simulink model "Reporting_assignment2"  (R2023b)
settings: Solver=VariableStepAuto  StartTime=0.0  StopTime=2.5  RelTol=1e-3
undefined symbols (not defined in the file): Bm, c1, delta, E, eta, Izzg1, J, Ke, Kp, Kt, La, m1, N, r1, Ra, Td, Ti
settings Model: SimulationMode=accelerator  Creator=Naoki  LastModifiedBy=Naoki

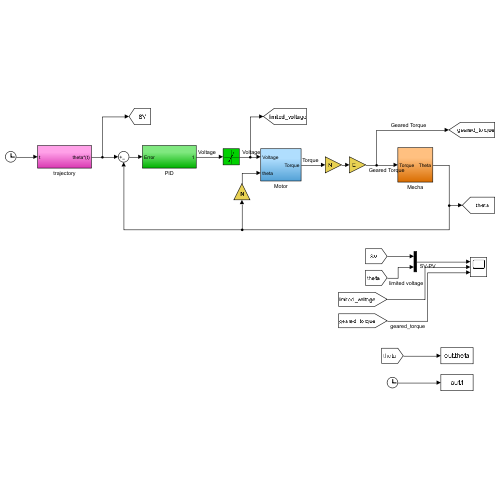
[thumbnail: Simulink's stored preview of the top-level diagram]
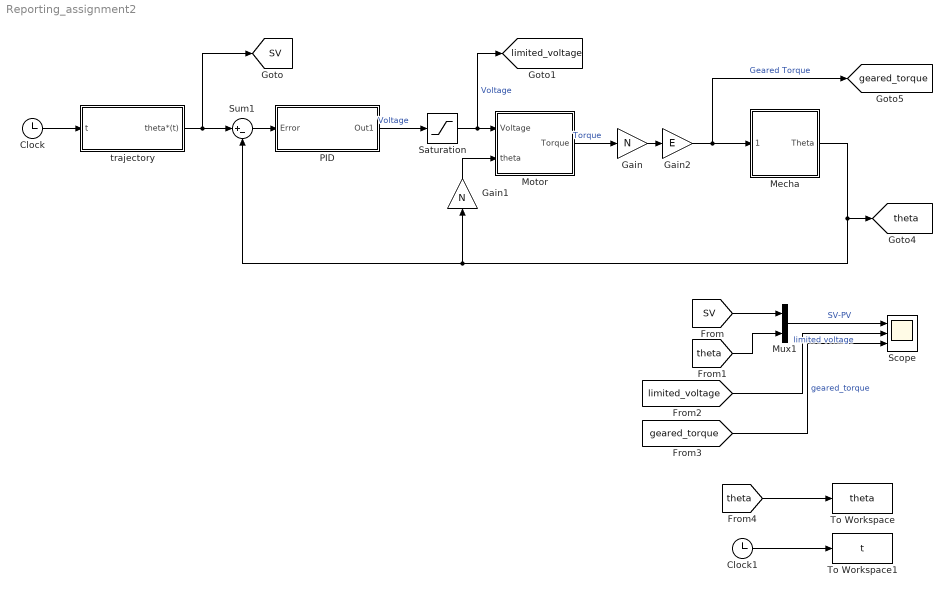
== system Reporting_assignment2 ==
  Clock : Clock
  Clock1 : Clock
  Gain : Gain  Gain=N
  Gain1 : Gain  Gain=N
  Gain2 : Gain  Gain=E
  Mecha : Subsystem
  Motor : Subsystem
  Mux1 : Mux  Inputs=2
  PID : Subsystem
  Saturation : Saturate  UpperLimit=20
  Scope : Scope  NumInputPorts=3
  Sum1 : Sum  Inputs=|+-
  To Workspace : ToWorkspace  VariableName=theta  SampleTime=0.1
  To Workspace1 : ToWorkspace  VariableName=t  SampleTime=0.1
  trajectory : Subsystem
  tag scope: SV=global, geared_torque=global, limited_voltage=global, theta=global
  wires:
  [theta] -> To Workspace/1
  Clock/1 -> trajectory/1(t)
  Clock1/1 -> To Workspace1/1
  Mux1/1 -> Scope/1  "SV-PV"
  [geared_torque] -> Scope/3  "geared_torque"
  [theta] -> Mux1/2
  PID/1(Out1) -> Saturation/1  "Voltage"
  Gain1/1 -> Motor/2(theta)
  Gain2/1 -> [geared_torque], Mecha/1(Torque)  "Geared Torque"
  Mecha/1(Theta) -> Sum1/2, Gain1/1, [theta]
  Gain/1 -> Gain2/1
  Saturation/1 -> [limited_voltage], Motor/1(Voltage)  "Voltage"
  [SV] -> Mux1/1
  Motor/1(Torque) -> Gain/1  "Torque"
  trajectory/1(theta*(t)) -> Sum1/1, [SV]
  Sum1/1 -> PID/1(Error)
  [limited_voltage] -> Scope/2  "limited voltage"

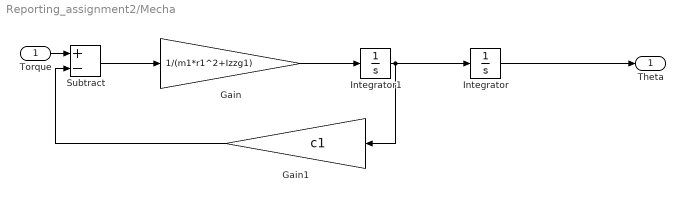
== system Reporting_assignment2/Mecha ==
  Torque : Inport
  Gain : Gain  Gain=1/(m1*r1^2+Izzg1)
  Gain1 : Gain  Gain=c1
  Integrator : Integrator
  Integrator1 : Integrator
  Subtract : Sum  Inputs=+-
  Theta : Outport
  wires:
  Integrator/1 -> Theta/1
  Integrator1/1 -> Gain1/1, Integrator/1
  Subtract/1 -> Gain/1
  Gain/1 -> Integrator1/1
  Torque/1 -> Subtract/1
  Gain1/1 -> Subtract/2

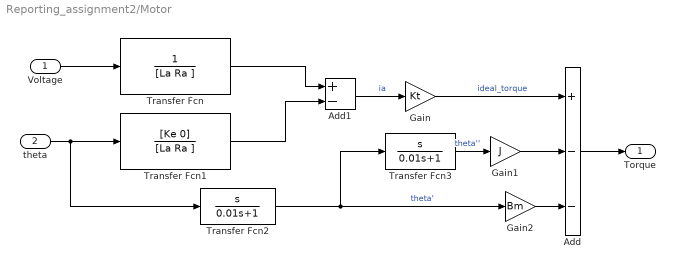
== system Reporting_assignment2/Motor ==
  Voltage : Inport
  theta : Inport  Port=2
  Add : Sum  Inputs=+--
  Add1 : Sum  Inputs=+-
  Gain : Gain  Gain=Kt
  Gain1 : Gain  Gain=J
  Gain2 : Gain  Gain=Bm
  Transfer Fcn : TransferFcn  Denominator=[La Ra ]
  Transfer Fcn1 : TransferFcn  Numerator=[Ke 0]  Denominator=[La Ra ]
  Transfer Fcn2 : TransferFcn  Numerator=[1 0]  Denominator=[0.01 1]
  Transfer Fcn3 : TransferFcn  Numerator=[1 0]  Denominator=[0.01 1]
  Torque : Outport
  wires:
  Transfer Fcn/1 -> Add1/1
  Transfer Fcn1/1 -> Add1/2
  Add1/1 -> Gain/1  "ia"
  Voltage/1 -> Transfer Fcn/1
  Gain/1 -> Add/1  "ideal_torque"
  theta/1 -> Transfer Fcn1/1, Transfer Fcn2/1
  Transfer Fcn3/1 -> Gain1/1  "theta''"
  Gain1/1 -> Add/2
  Gain2/1 -> Add/3
  Add/1 -> Torque/1
  Transfer Fcn2/1 -> Gain2/1, Transfer Fcn3/1  "theta'"

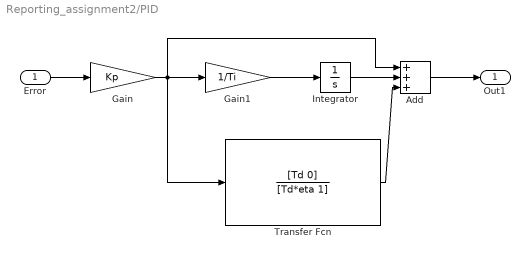
== system Reporting_assignment2/PID ==
  Error : Inport
  Add : Sum  Inputs=+++
  Gain : Gain  Gain=Kp
  Gain1 : Gain  Gain=1/Ti
  Integrator : Integrator
  Transfer Fcn : TransferFcn  Numerator=[Td 0]  Denominator=[Td*eta 1]
  Out1 : Outport
  wires:
  Add/1 -> Out1/1
  Integrator/1 -> Add/2
  Error/1 -> Gain/1
  Gain/1 -> Transfer Fcn/1, Add/1, Gain1/1
  Transfer Fcn/1 -> Add/3
  Gain1/1 -> Integrator/1

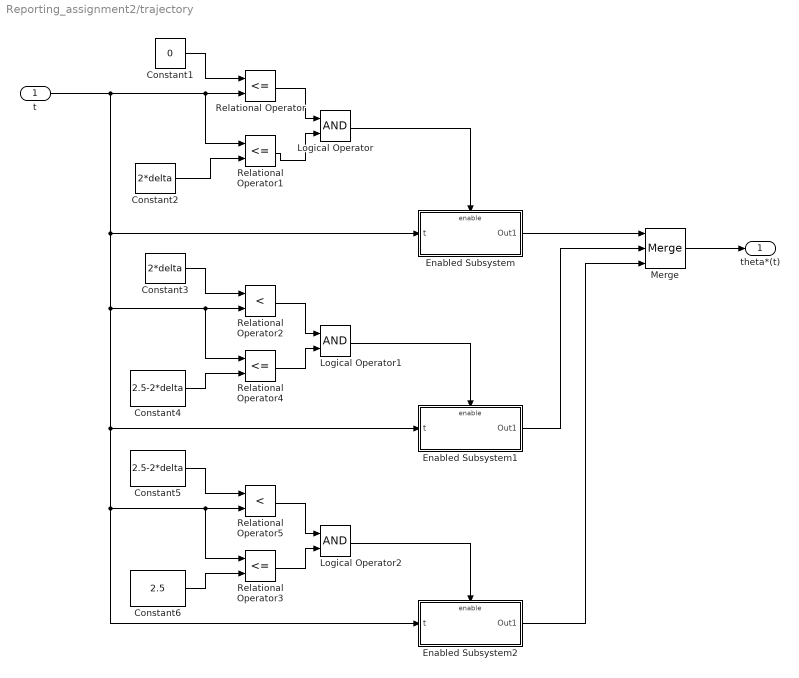
== system Reporting_assignment2/trajectory ==
  t : Inport
  Constant1 : Constant  Value=0
  Constant2 : Constant  Value=2*delta
  Constant3 : Constant  Value=2*delta
  Constant4 : Constant  Value=2.5-2*delta
  Constant5 : Constant  Value=2.5-2*delta
  Constant6 : Constant  Value=2.5
  Enabled Subsystem : Subsystem  TreatAsAtomicUnit=on
  Enabled Subsystem1 : Subsystem  TreatAsAtomicUnit=on
  Enabled Subsystem2 : Subsystem  TreatAsAtomicUnit=on
  Logical Operator : Logic  AllPortsSameDT=off  OutDataTypeStr=boolean
  Logical Operator1 : Logic  AllPortsSameDT=off  OutDataTypeStr=boolean
  Logical Operator2 : Logic  AllPortsSameDT=off  OutDataTypeStr=boolean
  Merge : Merge  Inputs=3
  Relational Operator{,1,3..4} (4 alike) : RelationalOperator  Operator=<=  OutDataTypeStr=boolean  InputSameDT=off
  Relational Operator2 : RelationalOperator  Operator=<  OutDataTypeStr=boolean  InputSameDT=off
  Relational Operator5 : RelationalOperator  Operator=<  OutDataTypeStr=boolean  InputSameDT=off
  theta*(t) : Outport
  wires:
  t/1 -> Relational Operator/2, Relational Operator1/1, Enabled Subsystem/1(t), Relational Operator2/2, Relational Operator4/1, Relational Operator5/2, Relational Operator3/1, Enabled Subsystem2/1(t), Enabled Subsystem1/1(t)
  Constant1/1 -> Relational Operator/1
  Relational Operator/1 -> Logical Operator/1
  Constant2/1 -> Relational Operator1/2
  Relational Operator1/1 -> Logical Operator/2
  Logical Operator/1 -> Enabled Subsystem/Enable
  Enabled Subsystem/1(Out1) -> Merge/1
  Merge/1 -> theta*(t)/1
  Constant3/1 -> Relational Operator2/1
  Relational Operator2/1 -> Logical Operator1/1
  Constant4/1 -> Relational Operator4/2
  Relational Operator4/1 -> Logical Operator1/2
  Enabled Subsystem1/1(Out1) -> Merge/2
  Logical Operator1/1 -> Enabled Subsystem1/Enable
  Constant5/1 -> Relational Operator5/1
  Relational Operator5/1 -> Logical Operator2/1
  Constant6/1 -> Relational Operator3/2
  Relational Operator3/1 -> Logical Operator2/2
  Enabled Subsystem2/1(Out1) -> Merge/3
  Logical Operator2/1 -> Enabled Subsystem2/Enable

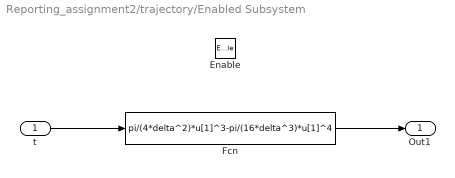
== system Reporting_assignment2/trajectory/Enabled Subsystem ==
  t : Inport
  Enable : EnablePort
  Fcn : Fcn  Expr=pi/(4*delta^2)*u[1]^3-pi/(16*delta^3)*u[1]^4
  Out1 : Outport
  wires:
  t/1 -> Fcn/1
  Fcn/1 -> Out1/1

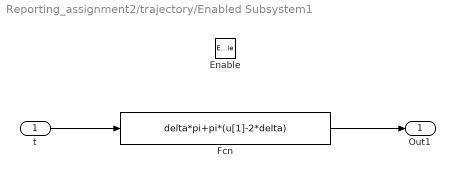
== system Reporting_assignment2/trajectory/Enabled Subsystem1 ==
  t : Inport
  Enable : EnablePort
  Fcn : Fcn  Expr=delta*pi+pi*(u[1]-2*delta)
  Out1 : Outport
  wires:
  Fcn/1 -> Out1/1
  t/1 -> Fcn/1

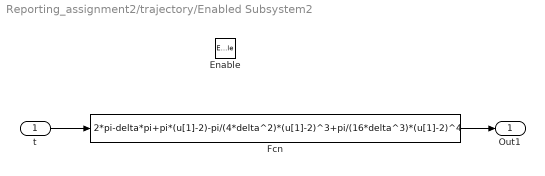
== system Reporting_assignment2/trajectory/Enabled Subsystem2 ==
  t : Inport
  Enable : EnablePort
  Fcn : Fcn  Expr=2*pi-delta*pi+pi*(u[1]-2)-pi/(4*delta^2)*(u[1]-2)^3+pi/(16*delta^3)*(u[1]-2)^4
  Out1 : Outport
  wires:
  t/1 -> Fcn/1
  Fcn/1 -> Out1/1
